simulink model "Trajectory_PID"  (R2024b)
settings: Solver=VariableStepAuto  StartTime=0.0  StopTime=10.0  RelTol=1e-3
libraries: slpidlib x4
settings Model: Creator=GH-X-ST  LastModifiedBy=GH-X-ST

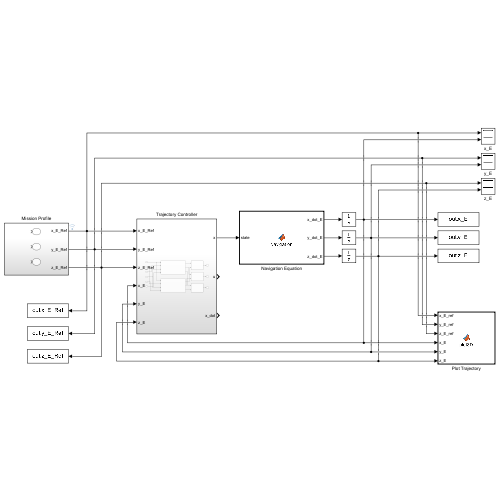
[thumbnail: Simulink's stored preview of the top-level diagram]
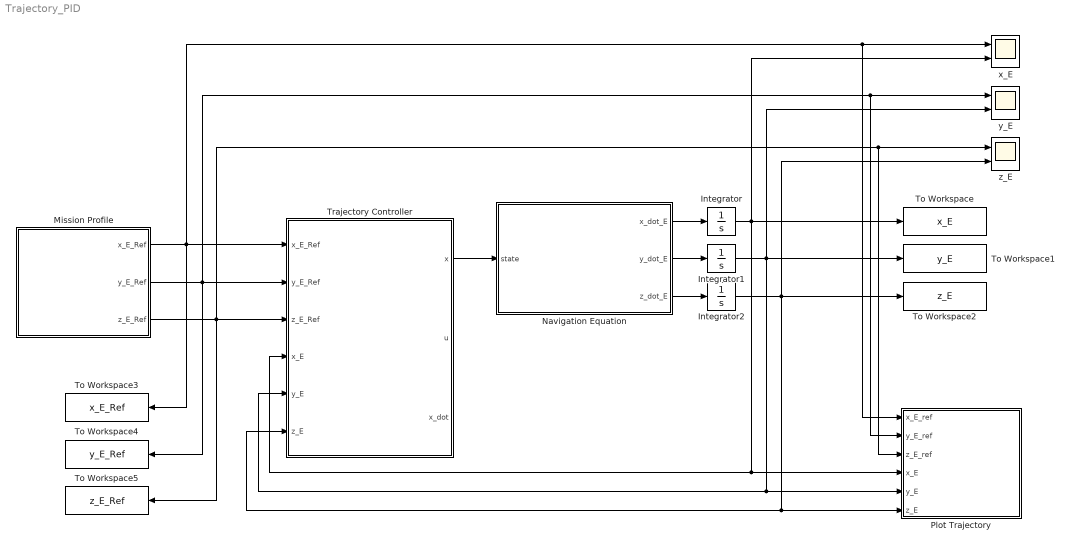
== system Trajectory_PID ==
  Integrator : Integrator
  Integrator1 : Integrator
  Integrator2 : Integrator
  Mission Profile : Subsystem
  Navigation Equation : MATLAB Function  TreatAsAtomicUnit=on
  Plot Trajectory : MATLAB Function  TreatAsAtomicUnit=on
  To Workspace : ToWorkspace  VariableName=x_E  SaveFormat=Timeseries  SampleTime=-1
  To Workspace1 : ToWorkspace  VariableName=y_E  SaveFormat=Timeseries  SampleTime=-1
  To Workspace2 : ToWorkspace  VariableName=z_E  SaveFormat=Timeseries  SampleTime=-1
  To Workspace3 : ToWorkspace  VariableName=x_E_Ref  SaveFormat=Timeseries  SampleTime=-1
  To Workspace4 : ToWorkspace  VariableName=y_E_Ref  SaveFormat=Timeseries  SampleTime=-1
  To Workspace5 : ToWorkspace  VariableName=z_E_Ref  SaveFormat=Timeseries  SampleTime=-1
  Trajectory Controller : Subsystem
  x_E : Scope  NumInputPorts=2
  y_E : Scope  NumInputPorts=2
  z_E : Scope  NumInputPorts=2
  wires:
  Navigation Equation/1(x_dot_E) -> Integrator/1
  Integrator/1 -> Trajectory Controller/4(x_E), Plot Trajectory/4(x_E), x_E/2, To Workspace/1
  Navigation Equation/2(y_dot_E) -> Integrator1/1
  Integrator1/1 -> Trajectory Controller/5(y_E), Plot Trajectory/5(y_E), y_E/2, To Workspace1/1
  Navigation Equation/3(z_dot_E) -> Integrator2/1
  Integrator2/1 -> Trajectory Controller/6(z_E), Plot Trajectory/6(z_E), z_E/2, To Workspace2/1
  Mission Profile/1(x_E_Ref) -> To Workspace3/1, Plot Trajectory/1(x_E_ref), x_E/1, Trajectory Controller/1(x_E_Ref)
  Trajectory Controller/1(x) -> Navigation Equation/1(state)
  Mission Profile/2(y_E_Ref) -> Plot Trajectory/2(y_E_ref), y_E/1, Trajectory Controller/2(y_E_Ref), To Workspace4/1
  Mission Profile/3(z_E_Ref) -> To Workspace5/1, Plot Trajectory/3(z_E_ref), z_E/1, Trajectory Controller/3(z_E_Ref)

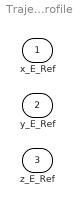
== system Trajectory_PID/Mission Profile ==
  x_E_Ref : Outport
  y_E_Ref : Outport  Port=2
  z_E_Ref : Outport  Port=3

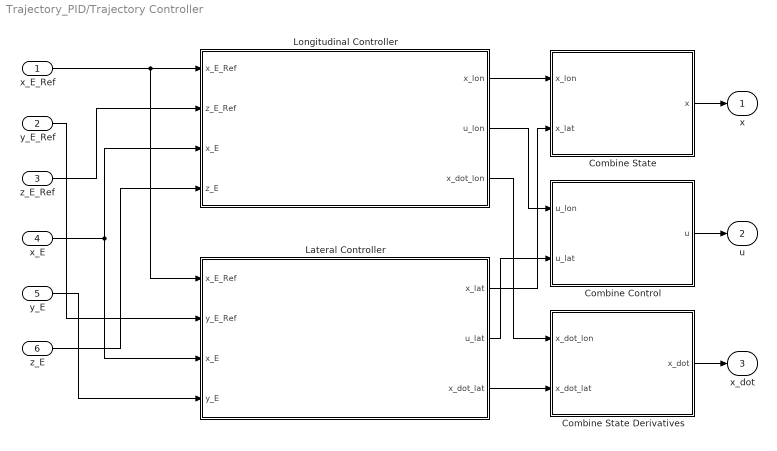
== system Trajectory_PID/Trajectory Controller ==
  x_E_Ref : Inport
  y_E_Ref : Inport  Port=2
  z_E_Ref : Inport  Port=3
  x_E : Inport  Port=4
  y_E : Inport  Port=5
  z_E : Inport  Port=6
  Combine Control : MATLAB Function  TreatAsAtomicUnit=on
  Combine State : MATLAB Function  TreatAsAtomicUnit=on
  Combine State Derivatives : MATLAB Function  TreatAsAtomicUnit=on
  Lateral Controller : Subsystem
  Longitudinal Controller : Subsystem
  x : Outport
  u : Outport  Port=2
  x_dot : Outport  Port=3
  wires:
  Combine State/1(x) -> x/1
  Combine Control/1(u) -> u/1
  Longitudinal Controller/2(u_lon) -> Combine Control/1(u_lon)
  Longitudinal Controller/1(x_lon) -> Combine State/1(x_lon)
  Lateral Controller/1(x_lat) -> Combine State/2(x_lat)
  Lateral Controller/2(u_lat) -> Combine Control/2(u_lat)
  Combine State Derivatives/1(x_dot) -> x_dot/1
  Lateral Controller/3(x_dot_lat) -> Combine State Derivatives/2(x_dot_lat)
  Longitudinal Controller/3(x_dot_lon) -> Combine State Derivatives/1(x_dot_lon)
  x_E_Ref/1 -> Lateral Controller/1(x_E_Ref), Longitudinal Controller/1(x_E_Ref)
  z_E_Ref/1 -> Longitudinal Controller/2(z_E_Ref)
  x_E/1 -> Lateral Controller/3(x_E), Longitudinal Controller/3(x_E)
  z_E/1 -> Longitudinal Controller/4(z_E)
  y_E_Ref/1 -> Lateral Controller/2(y_E_Ref)
  y_E/1 -> Lateral Controller/4(y_E)

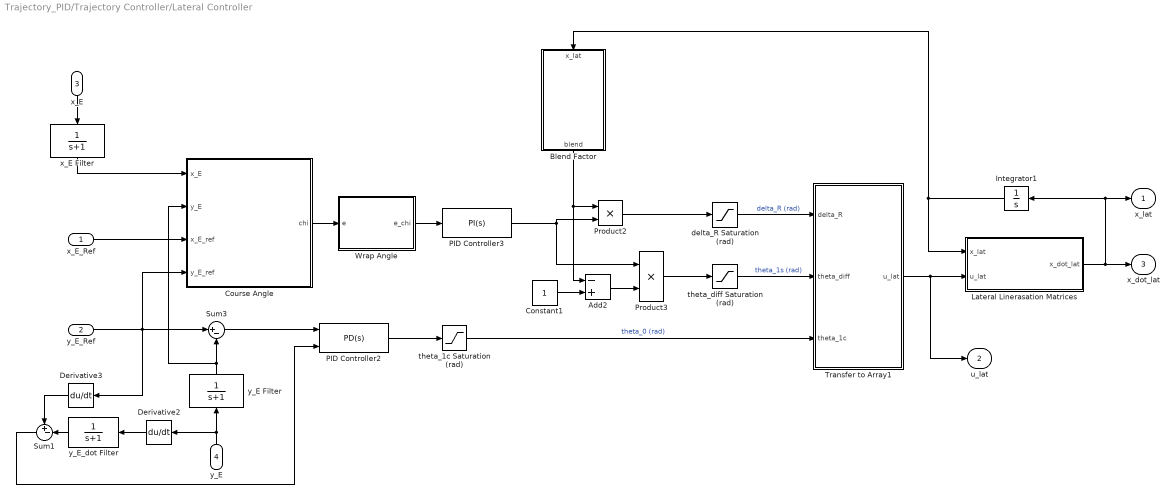
== system Trajectory_PID/Trajectory Controller/Lateral Controller ==
  x_E_Ref : Inport
  y_E_Ref : Inport  Port=2
  x_E : Inport  Port=3
  y_E : Inport  Port=4
  " Course Angle" : MATLAB Function  TreatAsAtomicUnit=on
  Add2 : Sum  Inputs=-+
  Blend Factor : MATLAB Function  TreatAsAtomicUnit=on
  Constant1 : Constant
  Derivative2 : Derivative  CoefficientInTFapproximation=0.05
  Derivative3 : Derivative  CoefficientInTFapproximation=0.05
  Integrator1 : Integrator
  Lateral Linerasation Matrices : MATLAB Function  TreatAsAtomicUnit=on
  PID Controller2 : slpidlib/PID Controller  Controller=PD  Form=Parallel  TimeDomain=Continuous-time  UseExternalTs=off  SampleTime=-1  IntegratorMethod=Forward Euler  FilterMethod=Forward Euler  ControllerParametersSource=internal  P=0.01  I=0.005  UseKiTs=off  D=0.005  UseExternalDerivativeSource=on  N=100  UseFilter=on  TunerSelectOption=Transfer Function Based (PID Tuner App)  InitialConditionSource=internal  InitialConditionForIntegrator=0  InitialConditionForFilter=0  DifferentiatorICPrevScaledInput=0  ExternalReset=none  TrackingMode=off  Kt=1  LimitOutput=on  SatLimitsSource=internal  UpperSaturationLimit=1  LowerSaturationLimit=-1  LinearizeAsGain=on  AntiWindupMode=none  Kb=1  LimitIntegrator=off  UpperIntegratorSaturationLimit=inf  LowerIntegratorSaturationLimit=-inf  POutMin=[]  POutMax=[]  IOutMin=[]  IOutMax=[]  DOutMin=[]  DOutMax=[]  NOutMin=[]  NOutMax=[]  SumOutMin=[]  SumOutMax=[]  SaturationOutMin=[]  SaturationOutMax=[]  PParamMin=[]  PParamMax=[]  IParamMin=[]  IParamMax=[]  DParamMin=[]  DParamMax=[]  NParamMin=[]  NParamMax=[]  KbParamMin=[]  KbParamMax=[]  KtParamMin=[]  KtParamMax=[]  KbOutMin=[]  KbOutMax=[]  KtOutMin=[]  KtOutMax=[]  IntegratorOutMin=[]  IntegratorOutMax=[]  FilterOutMin=[]  FilterOutMax=[]  SumI1OutMin=[]  SumI1OutMax=[]  SumI2OutMin=[]  SumI2OutMax=[]  SumI3OutMin=[]  SumI3OutMax=[]  SumI4OutMin=[]  SumI4OutMax=[]  SumDOutMin=[]  SumDOutMax=[]  DifferentiatorOutMin=[]  DifferentiatorOutMax=[]  FilterDiffOutCoefMin=[]  FilterDiffOutCoefMax=[]  ReciprocalOutMin=[]  ReciprocalOutMax=[]  SumDenOutMin=[]  SumDenOutMax=[]  SumNumOutMin=[]  SumNumOutMax=[]  DivideOutMin=[]  DivideOutMax=[]  UdiffTsProdOutMin=[]  UdiffTsProdOutMax=[]  NTsProdOutMin=[]  NTsProdOutMax=[]  UintegralTsProdOutMin=[]  UintegralTsProdOutMax=[]  UngainTsProdOutMin=[]  UngainTsProdOutMax=[]  ClampingZeroOutDataTypeStr=Inherit: Inherit via back propagation  ClampingZeroOutMin=[]  ClampingZeroOutMax=[]  FilterDenConstantOutDataTypeStr=Inherit: Inherit via back propagation  FilterDenConstantOutMin=[]  FilterDenConstantOutMax=[]  PCopyOutDataTypeStr=Inherit: Inherit via back propagation  PCopyOutMin=[]  PCopyOutMax=[]  NCopyOutDataTypeStr=Inherit: Inherit via back propagation  NCopyOutMin=[]  NCopyOutMax=[]  IntegratorContinuousStateAttributes=''  IntegratorStateMustResolveToSignalObject=off  IntegratorRTWStateStorageClass=Auto  FilterContinuousStateAttributes=''  FilterStateMustResolveToSignalObject=off  FilterRTWStateStorageClass=Auto  ParallelPVariant=InternalParameters  IdealPVariant=Disabled  IVariant=Disabled  DVariant=InternalParameters  IntegratorVariant=Disabled  SatVariant=Enabled  AWVariant=Disabled  PCopyVariant=Disabled  TRVariant=Disabled  FdbkBlocksVariant=Forward  IdealPFdbkVariant=Disabled  SatFdbkVariant=Disabled  DerivativeFilterVariant=ContFilterOnly  NVariant=InternalParameters  NCopyVariant=Disabled  FilterICVariant=InternalICsFilter  IntegratorICVariant=Disabled  ExternalResetVariant=Disabled  TRSumVariant=Passthrough  SumFdbkVariant=Disabled  SumVariant=Sum_PD  TsampFilterVariant=InternalTs  TsampNgainVariant=Passthrough  TsampIntegralVariant=Disabled_SignalSpec  ExternalSaturationOutDataTypeStr=Inherit: Same as second input  DerivativeSourceVariant=ExternalYdot  PreIntVariant=InternalPreInt
  PID Controller3 : slpidlib/PID Controller  Controller=PI  Form=Parallel  TimeDomain=Continuous-time  UseExternalTs=off  SampleTime=-1  IntegratorMethod=Forward Euler  FilterMethod=Forward Euler  ControllerParametersSource=internal  P=0.01  I=0.005  UseKiTs=off  D=0.005  UseExternalDerivativeSource=off  N=100  UseFilter=on  TunerSelectOption=Transfer Function Based (PID Tuner App)  InitialConditionSource=internal  InitialConditionForIntegrator=0  InitialConditionForFilter=0  DifferentiatorICPrevScaledInput=0  ExternalReset=none  TrackingMode=off  Kt=1  LimitOutput=on  SatLimitsSource=internal  UpperSaturationLimit=1  LowerSaturationLimit=-1  LinearizeAsGain=on  AntiWindupMode=none  Kb=1  LimitIntegrator=off  UpperIntegratorSaturationLimit=inf  LowerIntegratorSaturationLimit=-inf  POutMin=[]  POutMax=[]  IOutMin=[]  IOutMax=[]  DOutMin=[]  DOutMax=[]  NOutMin=[]  NOutMax=[]  SumOutMin=[]  SumOutMax=[]  SaturationOutMin=[]  SaturationOutMax=[]  PParamMin=[]  PParamMax=[]  IParamMin=[]  IParamMax=[]  DParamMin=[]  DParamMax=[]  NParamMin=[]  NParamMax=[]  KbParamMin=[]  KbParamMax=[]  KtParamMin=[]  KtParamMax=[]  KbOutMin=[]  KbOutMax=[]  KtOutMin=[]  KtOutMax=[]  IntegratorOutMin=[]  IntegratorOutMax=[]  FilterOutMin=[]  FilterOutMax=[]  SumI1OutMin=[]  SumI1OutMax=[]  SumI2OutMin=[]  SumI2OutMax=[]  SumI3OutMin=[]  SumI3OutMax=[]  SumI4OutMin=[]  SumI4OutMax=[]  SumDOutMin=[]  SumDOutMax=[]  DifferentiatorOutMin=[]  DifferentiatorOutMax=[]  FilterDiffOutCoefMin=[]  FilterDiffOutCoefMax=[]  ReciprocalOutMin=[]  ReciprocalOutMax=[]  SumDenOutMin=[]  SumDenOutMax=[]  SumNumOutMin=[]  SumNumOutMax=[]  DivideOutMin=[]  DivideOutMax=[]  UdiffTsProdOutMin=[]  UdiffTsProdOutMax=[]  NTsProdOutMin=[]  NTsProdOutMax=[]  UintegralTsProdOutMin=[]  UintegralTsProdOutMax=[]  UngainTsProdOutMin=[]  UngainTsProdOutMax=[]  ClampingZeroOutDataTypeStr=Inherit: Inherit via back propagation  ClampingZeroOutMin=[]  ClampingZeroOutMax=[]  FilterDenConstantOutDataTypeStr=Inherit: Inherit via back propagation  FilterDenConstantOutMin=[]  FilterDenConstantOutMax=[]  PCopyOutDataTypeStr=Inherit: Inherit via back propagation  PCopyOutMin=[]  PCopyOutMax=[]  NCopyOutDataTypeStr=Inherit: Inherit via back propagation  NCopyOutMin=[]  NCopyOutMax=[]  IntegratorContinuousStateAttributes=''  IntegratorStateMustResolveToSignalObject=off  IntegratorRTWStateStorageClass=Auto  FilterContinuousStateAttributes=''  FilterStateMustResolveToSignalObject=off  FilterRTWStateStorageClass=Auto  ParallelPVariant=InternalParameters  IdealPVariant=Disabled  IVariant=InternalParameters  DVariant=Disabled  IntegratorVariant=Continuous  SatVariant=Enabled  AWVariant=Passthrough  PCopyVariant=Disabled  TRVariant=Disabled  FdbkBlocksVariant=Forward  IdealPFdbkVariant=Disabled  SatFdbkVariant=Disabled  DerivativeFilterVariant=Disabled  NVariant=Disabled  NCopyVariant=Disabled_SignalSpec  FilterICVariant=Disabled  IntegratorICVariant=InternalICs  ExternalResetVariant=Disabled  TRSumVariant=Passthrough  SumFdbkVariant=Disabled  SumVariant=Sum_PI  TsampFilterVariant=InternalTs  TsampNgainVariant=Passthrough  TsampIntegralVariant=Disabled_SignalSpec  ExternalSaturationOutDataTypeStr=Inherit: Same as second input  DerivativeSourceVariant=Disabled  PreIntVariant=InternalPreInt
  Product2 : Product
  Product3 : Product
  Sum1 : Sum  Inputs=+-|
  Sum3 : Sum  Inputs=|+-
  Transfer to Array1 : MATLAB Function  TreatAsAtomicUnit=on
  Wrap Angle : MATLAB Function  TreatAsAtomicUnit=on
  delta_R Saturation (rad) : Saturate
  theta_1c Saturation (rad) : Saturate
  theta_diff Saturation (rad) : Saturate
  x_E Filter : TransferFcn  Denominator=[1 1]
  y_E Filter : TransferFcn  Denominator=[1 1]
  y_E_dot Filter : TransferFcn  Denominator=[1 1]
  x_lat : Outport
  u_lat : Outport  Port=2
  x_dot_lat : Outport  Port=3
  wires:
  y_E/1 -> y_E Filter/1, Derivative2/1
  y_E Filter/1 -> Sum3/2, " Course Angle"/2(y_E)
  y_E_Ref/1 -> Derivative3/1, " Course Angle"/4(y_E_ref), Sum3/1
  Sum3/1 -> PID Controller2/1
  PID Controller2/1 -> theta_1c Saturation (rad)/1
  theta_1c Saturation (rad)/1 -> Transfer to Array1/3(theta_1c)  "theta_0 (rad)"
  Transfer to Array1/1(u_lat) -> u_lat/1, Lateral Linerasation Matrices/2(u_lat)
  Lateral Linerasation Matrices/1(x_dot_lat) -> Integrator1/1, x_lat/1, x_dot_lat/1
  Integrator1/1 -> Lateral Linerasation Matrices/1(x_lat), Blend Factor/1(x_lat)
  x_E_Ref/1 -> " Course Angle"/3(x_E_ref)
  " Course Angle"/1(chi) -> Wrap Angle/1(e)
  Wrap Angle/1(e_chi) -> PID Controller3/1
  PID Controller3/1 -> Product2/2, Product3/1
  Blend Factor/1(blend) -> Add2/1, Product2/1
  Constant1/1 -> Add2/2
  Add2/1 -> Product3/2
  Product3/1 -> theta_diff Saturation (rad)/1
  theta_diff Saturation (rad)/1 -> Transfer to Array1/2(theta_diff)  "theta_1s (rad)"
  Product2/1 -> delta_R Saturation (rad)/1
  delta_R Saturation (rad)/1 -> Transfer to Array1/1(delta_R)  "delta_R (rad)"
  x_E/1 -> x_E Filter/1
  x_E Filter/1 -> " Course Angle"/1(x_E)
  Derivative2/1 -> y_E_dot Filter/1
  Derivative3/1 -> Sum1/1
  y_E_dot Filter/1 -> Sum1/2
  Sum1/1 -> PID Controller2/2

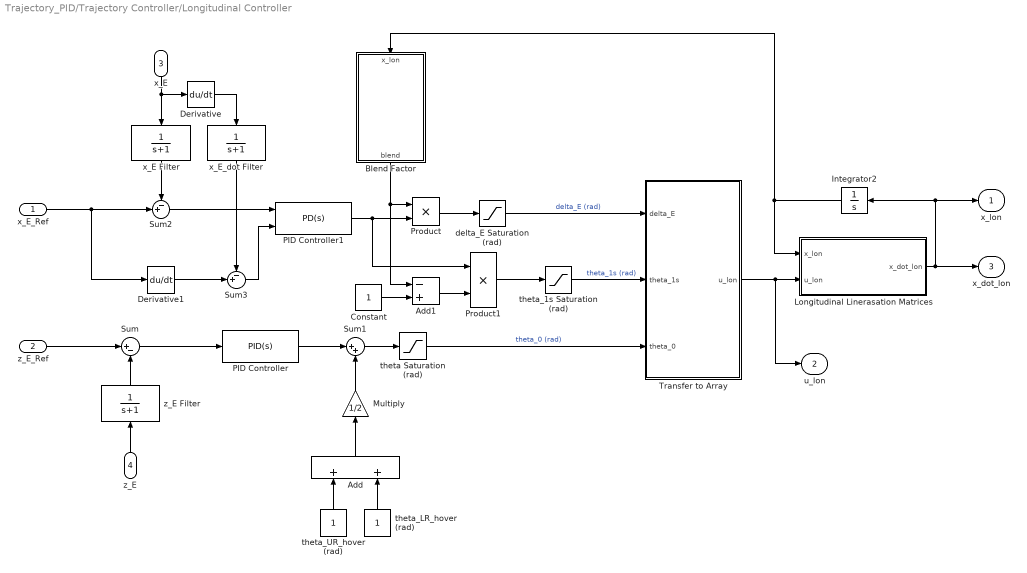
== system Trajectory_PID/Trajectory Controller/Longitudinal Controller ==
  x_E_Ref : Inport
  z_E_Ref : Inport  Port=2
  x_E : Inport  Port=3
  z_E : Inport  Port=4
  Add : Sum
  Add1 : Sum  Inputs=-+
  Blend Factor : MATLAB Function  TreatAsAtomicUnit=on
  Constant : Constant
  Derivative : Derivative  CoefficientInTFapproximation=0.05
  Derivative1 : Derivative  CoefficientInTFapproximation=0.05
  Integrator2 : Integrator
  Longitudinal Linerasation Matrices : MATLAB Function  TreatAsAtomicUnit=on
  Multiply : Gain  Gain=1/2
  PID Controller : slpidlib/PID Controller  Controller=PID  Form=Parallel  TimeDomain=Continuous-time  UseExternalTs=off  SampleTime=-1  IntegratorMethod=Forward Euler  FilterMethod=Forward Euler  ControllerParametersSource=internal  P=0.01  I=0.005  UseKiTs=off  D=0.005  UseExternalDerivativeSource=off  N=100  UseFilter=on  TunerSelectOption=Transfer Function Based (PID Tuner App)  InitialConditionSource=internal  InitialConditionForIntegrator=0  InitialConditionForFilter=0  DifferentiatorICPrevScaledInput=0  ExternalReset=none  TrackingMode=off  Kt=1  LimitOutput=on  SatLimitsSource=internal  UpperSaturationLimit=1  LowerSaturationLimit=-1  LinearizeAsGain=on  AntiWindupMode=none  Kb=1  LimitIntegrator=off  UpperIntegratorSaturationLimit=inf  LowerIntegratorSaturationLimit=-inf  POutMin=[]  POutMax=[]  IOutMin=[]  IOutMax=[]  DOutMin=[]  DOutMax=[]  NOutMin=[]  NOutMax=[]  SumOutMin=[]  SumOutMax=[]  SaturationOutMin=[]  SaturationOutMax=[]  PParamMin=[]  PParamMax=[]  IParamMin=[]  IParamMax=[]  DParamMin=[]  DParamMax=[]  NParamMin=[]  NParamMax=[]  KbParamMin=[]  KbParamMax=[]  KtParamMin=[]  KtParamMax=[]  KbOutMin=[]  KbOutMax=[]  KtOutMin=[]  KtOutMax=[]  IntegratorOutMin=[]  IntegratorOutMax=[]  FilterOutMin=[]  FilterOutMax=[]  SumI1OutMin=[]  SumI1OutMax=[]  SumI2OutMin=[]  SumI2OutMax=[]  SumI3OutMin=[]  SumI3OutMax=[]  SumI4OutMin=[]  SumI4OutMax=[]  SumDOutMin=[]  SumDOutMax=[]  DifferentiatorOutMin=[]  DifferentiatorOutMax=[]  FilterDiffOutCoefMin=[]  FilterDiffOutCoefMax=[]  ReciprocalOutMin=[]  ReciprocalOutMax=[]  SumDenOutMin=[]  SumDenOutMax=[]  SumNumOutMin=[]  SumNumOutMax=[]  DivideOutMin=[]  DivideOutMax=[]  UdiffTsProdOutMin=[]  UdiffTsProdOutMax=[]  NTsProdOutMin=[]  NTsProdOutMax=[]  UintegralTsProdOutMin=[]  UintegralTsProdOutMax=[]  UngainTsProdOutMin=[]  UngainTsProdOutMax=[]  ClampingZeroOutDataTypeStr=Inherit: Inherit via back propagation  ClampingZeroOutMin=[]  ClampingZeroOutMax=[]  FilterDenConstantOutDataTypeStr=Inherit: Inherit via back propagation  FilterDenConstantOutMin=[]  FilterDenConstantOutMax=[]  PCopyOutDataTypeStr=Inherit: Inherit via back propagation  PCopyOutMin=[]  PCopyOutMax=[]  NCopyOutDataTypeStr=Inherit: Inherit via back propagation  NCopyOutMin=[]  NCopyOutMax=[]  IntegratorContinuousStateAttributes=''  IntegratorStateMustResolveToSignalObject=off  IntegratorRTWStateStorageClass=Auto  FilterContinuousStateAttributes=''  FilterStateMustResolveToSignalObject=off  FilterRTWStateStorageClass=Auto  ParallelPVariant=InternalParameters  IdealPVariant=Disabled  IVariant=InternalParameters  DVariant=InternalParameters  IntegratorVariant=Continuous  SatVariant=Enabled  AWVariant=Passthrough  PCopyVariant=Disabled  TRVariant=Disabled  FdbkBlocksVariant=Forward  IdealPFdbkVariant=Disabled  SatFdbkVariant=Disabled  DerivativeFilterVariant=ContFilter  NVariant=InternalParameters  NCopyVariant=Disabled  FilterICVariant=InternalICsFilter  IntegratorICVariant=InternalICs  ExternalResetVariant=Disabled  TRSumVariant=Passthrough  SumFdbkVariant=Disabled  SumVariant=Sum_PID  TsampFilterVariant=InternalTs  TsampNgainVariant=Passthrough  TsampIntegralVariant=Disabled_SignalSpec  ExternalSaturationOutDataTypeStr=Inherit: Same as second input  DerivativeSourceVariant=ErrorSignal  PreIntVariant=InternalPreInt
  PID Controller1 : slpidlib/PID Controller  Controller=PD  Form=Parallel  TimeDomain=Continuous-time  UseExternalTs=off  SampleTime=-1  IntegratorMethod=Forward Euler  FilterMethod=Forward Euler  ControllerParametersSource=internal  P=0.01  I=0.005  UseKiTs=off  D=0.005  UseExternalDerivativeSource=on  N=100  UseFilter=on  TunerSelectOption=Transfer Function Based (PID Tuner App)  InitialConditionSource=internal  InitialConditionForIntegrator=0  InitialConditionForFilter=0  DifferentiatorICPrevScaledInput=0  ExternalReset=none  TrackingMode=off  Kt=1  LimitOutput=on  SatLimitsSource=internal  UpperSaturationLimit=1  LowerSaturationLimit=-1  LinearizeAsGain=on  AntiWindupMode=none  Kb=1  LimitIntegrator=off  UpperIntegratorSaturationLimit=inf  LowerIntegratorSaturationLimit=-inf  POutMin=[]  POutMax=[]  IOutMin=[]  IOutMax=[]  DOutMin=[]  DOutMax=[]  NOutMin=[]  NOutMax=[]  SumOutMin=[]  SumOutMax=[]  SaturationOutMin=[]  SaturationOutMax=[]  PParamMin=[]  PParamMax=[]  IParamMin=[]  IParamMax=[]  DParamMin=[]  DParamMax=[]  NParamMin=[]  NParamMax=[]  KbParamMin=[]  KbParamMax=[]  KtParamMin=[]  KtParamMax=[]  KbOutMin=[]  KbOutMax=[]  KtOutMin=[]  KtOutMax=[]  IntegratorOutMin=[]  IntegratorOutMax=[]  FilterOutMin=[]  FilterOutMax=[]  SumI1OutMin=[]  SumI1OutMax=[]  SumI2OutMin=[]  SumI2OutMax=[]  SumI3OutMin=[]  SumI3OutMax=[]  SumI4OutMin=[]  SumI4OutMax=[]  SumDOutMin=[]  SumDOutMax=[]  DifferentiatorOutMin=[]  DifferentiatorOutMax=[]  FilterDiffOutCoefMin=[]  FilterDiffOutCoefMax=[]  ReciprocalOutMin=[]  ReciprocalOutMax=[]  SumDenOutMin=[]  SumDenOutMax=[]  SumNumOutMin=[]  SumNumOutMax=[]  DivideOutMin=[]  DivideOutMax=[]  UdiffTsProdOutMin=[]  UdiffTsProdOutMax=[]  NTsProdOutMin=[]  NTsProdOutMax=[]  UintegralTsProdOutMin=[]  UintegralTsProdOutMax=[]  UngainTsProdOutMin=[]  UngainTsProdOutMax=[]  ClampingZeroOutDataTypeStr=Inherit: Inherit via back propagation  ClampingZeroOutMin=[]  ClampingZeroOutMax=[]  FilterDenConstantOutDataTypeStr=Inherit: Inherit via back propagation  FilterDenConstantOutMin=[]  FilterDenConstantOutMax=[]  PCopyOutDataTypeStr=Inherit: Inherit via back propagation  PCopyOutMin=[]  PCopyOutMax=[]  NCopyOutDataTypeStr=Inherit: Inherit via back propagation  NCopyOutMin=[]  NCopyOutMax=[]  IntegratorContinuousStateAttributes=''  IntegratorStateMustResolveToSignalObject=off  IntegratorRTWStateStorageClass=Auto  FilterContinuousStateAttributes=''  FilterStateMustResolveToSignalObject=off  FilterRTWStateStorageClass=Auto  ParallelPVariant=InternalParameters  IdealPVariant=Disabled  IVariant=Disabled  DVariant=InternalParameters  IntegratorVariant=Disabled  SatVariant=Enabled  AWVariant=Disabled  PCopyVariant=Disabled  TRVariant=Disabled  FdbkBlocksVariant=Forward  IdealPFdbkVariant=Disabled  SatFdbkVariant=Disabled  DerivativeFilterVariant=ContFilterOnly  NVariant=InternalParameters  NCopyVariant=Disabled  FilterICVariant=InternalICsFilter  IntegratorICVariant=Disabled  ExternalResetVariant=Disabled  TRSumVariant=Passthrough  SumFdbkVariant=Disabled  SumVariant=Sum_PD  TsampFilterVariant=InternalTs  TsampNgainVariant=Passthrough  TsampIntegralVariant=Disabled_SignalSpec  ExternalSaturationOutDataTypeStr=Inherit: Same as second input  DerivativeSourceVariant=ExternalYdot  PreIntVariant=InternalPreInt
  Product : Product
  Product1 : Product
  Sum : Sum  Inputs=|+-
  Sum1 : Sum  Inputs=|++
  Sum2 : Sum  Inputs=-+|
  Sum3 : Sum  Inputs=-+|
  Transfer to Array : MATLAB Function  TreatAsAtomicUnit=on
  delta_E Saturation (rad) : Saturate
  theta Saturation (rad) : Saturate
  theta_1s Saturation (rad) : Saturate
  theta_LR_hover (rad) : Constant
  theta_UR_hover (rad) : Constant
  x_E Filter : TransferFcn  Denominator=[1 1]
  x_E_dot Filter : TransferFcn  Denominator=[1 1]
  z_E Filter : TransferFcn  Denominator=[1 1]
  x_lon : Outport
  u_lon : Outport  Port=2
  x_dot_lon : Outport  Port=3
  wires:
  z_E_Ref/1 -> Sum/1
  Sum/1 -> PID Controller/1
  PID Controller/1 -> Sum1/1
  Sum1/1 -> theta Saturation (rad)/1
  theta_UR_hover (rad)/1 -> Add/1
  theta_LR_hover (rad)/1 -> Add/2
  Multiply/1 -> Sum1/2
  Add/1 -> Multiply/1
  theta Saturation (rad)/1 -> Transfer to Array/3(theta_0)  "theta_0 (rad)"
  z_E Filter/1 -> Sum/2
  z_E/1 -> z_E Filter/1
  x_E/1 -> Derivative/1, x_E Filter/1
  x_E_Ref/1 -> Derivative1/1, Sum2/2
  Sum2/1 -> PID Controller1/1
  Integrator2/1 -> Longitudinal Linerasation Matrices/1(x_lon), Blend Factor/1(x_lon)
  Longitudinal Linerasation Matrices/1(x_dot_lon) -> Integrator2/1, x_lon/1, x_dot_lon/1
  Blend Factor/1(blend) -> Add1/1, Product/1
  PID Controller1/1 -> Product1/1, Product/2
  Product/1 -> delta_E Saturation (rad)/1
  delta_E Saturation (rad)/1 -> Transfer to Array/1(delta_E)  "delta_E (rad)"
  Constant/1 -> Add1/2
  Add1/1 -> Product1/2
  Product1/1 -> theta_1s Saturation (rad)/1
  theta_1s Saturation (rad)/1 -> Transfer to Array/2(theta_1s)  "theta_1s (rad)"
  Transfer to Array/1(u_lon) -> u_lon/1, Longitudinal Linerasation Matrices/2(u_lon)
  Derivative/1 -> x_E_dot Filter/1
  x_E Filter/1 -> Sum2/1
  Derivative1/1 -> Sum3/2
  x_E_dot Filter/1 -> Sum3/1
  Sum3/1 -> PID Controller1/2

== matlab function Trajectory_PID/Trajectory Controller/Lateral Controller/Lateral Linerasation Matrices ==
  data: x_dot_lat output; x_lat input; u_lat input
function x_dot_lat = Lon_linear(x_lat, u_lat)
% Author:
%   Hanchen Li (hl3422@ic.ac.uk)
%
% Inputs:
%   x_lat     - [v, p, r, phi, psi]
%   v         - Lateral velocity (m/s)
%   p         - Roll rate (rad/s)
%   r         - Yaw rate (rad/s)
%   phi       - Euler roll angle (rad)
%   psi       - Euler yaw angle (rad)
%
%   u_lat      - [theta_diff, theta_1c, delta_R]
%   theta_diff - Rotor collective difference (rad)
%   theta_1c   - Lateral cyclic (rad)
%   delta_R    - Rudder deflection (rad)
%
% Outputs:
%   x_dot_lat     - [v_dot, p_dot, r_dot, phi_dot, psi_dot]

%% 0 Extract Parameters
v          = x_lat(1);
p          = x_lat(2);
r          = x_lat(3);
phi        = x_lat(4);
psi        = x_lat(5);

theta_diff = u_lat(1);
theta_1c   = u_lat(2);
delta_R    = u_lat(3);

%% 1 Decide blend factor

if v = 0

    x_dot_lat = ;

else
    
    x_dot_lat = ;

end

end

== matlab function Trajectory_PID/Trajectory Controller/Lateral Controller/Blend Factor ==
  data: blend output; x_lat input
function blend = Blend_yaw(x_lat)
% Author:
%   Hanchen Li (hl3422@ic.ac.uk)
%
% Inputs:
%   x_lat     - [v, p, r, phi, psi]
%   v         - Lateral velocity (m/s)
%   p         - Roll rate (rad/s)
%   r         - Yaw rate (rad/s)
%   phi       - Euler roll angle (rad)
%   psi       - Euler yaw angle (rad)
%
% Outputs:
%   blend     - blend factor

%% 0 Extract Parameters

v   = x_lat(1);
p   = x_lat(2);
r   = x_lat(3);
phi = x_lat(4);
psi = x_lat(5);

%% 1 Decide blend factor

if abs(v) < 1e-4

    blend = 0;

elseif abs(v) < 20

    blend = u / 20;

else

    blend = 1;

end

end

== matlab function Trajectory_PID/Trajectory Controller/Lateral Controller/Wrap Angle ==
  data: e_chi output; e input
function e_chi = Wrap_Pi(e)
% Author:
%   Hanchen Li (hl3422@ic.ac.uk)
%
% Inputs:
%   chi
%
% Outputs:
%   e_chi

e_chi = mod(chi + pi, 2 * pi) - pi;

end

== matlab function Trajectory_PID/Plot Trajectory ==
  data: x_E_ref input; y_E_ref input; z_E_ref input; x_E input; y_E input; z_E input
function plot3D(x_E_ref, y_E_ref, z_E_ref, x_E, y_E, z_E)
% Author:
%   Hanchen Li (hl3422@ic.ac.uk)
%
% Inputs:
%   x_E_ref   - Distance in the Earth x-direction (m/s)
%   x_E_ref   - Distance in the Earth x-direction (m/s)
%   x_E_ref   - Distance in the Earth x-direction (m/s)
%   x_E       - Distance in the Earth x-direction (m/s)
%   x_E       - Distance in the Earth x-direction (m/s)
%   x_E       - Distance in the Earth x-direction (m/s)
%
% Outputs:
%   Real time 3D trajectory plot

% Persistent line objects for plotting
persistent refLine actLine firstRun

% Initialization (on first call)
if isempty(firstRun)
    
    figure(1); clf;
    refLine = animatedline('Color', [0/255 0/255 128/255], 'LineStyle', '--', 'LineWidth', 1.5, 'DisplayName', 'Reference');
    actLine = animatedline('Color', [220/255 20/255 60/255], 'LineStyle', '-',  'LineWidth', 1.5, 'DisplayName', 'Actual');
    xlabel('x_E'); ylabel('y_E'); zlabel('z_E');
    title('HALO 3-D trajectory plot.');
    grid on;
    view(3);
    legend show;
    axis equal;
    hold on;
    firstRun = true;
end

% Add new points
addpoints(refLine, x_ref, y_ref, z_ref);
addpoints(actLine, x, y, z);
    
% Update plot
drawnow limitrate;

end

== matlab function Trajectory_PID/Navigation Equation ==
  data: x_dot_E output; y_dot_E output; z_dot_E output; state input
function [x_dot_E, y_dot_E, z_dot_E] = Navigation(state)
% Author:
%   Hanchen Li (hl3422@ic.ac.uk)
%
% Inputs:
%   state     - [u, v, w, p, q, r, phi, theta, psi]
%   u         - Forward velocity (m/s)
%   v         - Lateral velocity (m/s)
%   w         - Vertical velocity (m/s)
%   p         - Roll rate (rad/s)
%   q         - Pitch rate (rad/s)
%   r         - Yaw rate (rad/s)
%   phi       - Euler roll angle (rad)
%   theta     - Euler pitch angle (rad)
%   psi       - Euler yaw angle (rad)
%
% Outputs:
%   x_dot_E   - Velocity in the Earth x-direction (m/s)
%   y_dot_E   - Velocity in the Earth y-direction (m/s)
%   z_dot_E   - Velocity in the Earth z-direction (m/s)

%% 0 Basic Parameters

% 0.1 Extract parameters
% state - [u, v, w, p, q, r, phi, theta, psi]
u = state(1);
v = state(2);
w = state(3);
p = state(4);
q = state(5);
r = state(6);
phi = state(7);
theta = state(8);
psi = state(9);

% 0.2 Compute trigonometric values
cphi = cos(phi);
sphi = sin(phi);
ctheta = cos(theta);
stheta = sin(theta);
cpsi = cos(psi);
spsi = sin(psi);

% 0.3 Transformation matrix from body to inertial frame
T = [...
     ctheta * cpsi, sphi * stheta * cpsi - cphi * spsi, cphi * stheta * cpsi + sphi * spsi;
     ctheta * spsi, sphi * stheta * spsi + cphi * cpsi, cphi * stheta * spsi - sphi * cpsi;
     -stheta      , sphi * ctheta                     , cphi * ctheta];

%% 1 Calculation
% 1.1 Body velocity vector
V_body = [u; v; w];

% 1.2 Compute inertial velocity
V_inertial = T * V_body;

% 1.3 Output
x_dot_E = V_inertial(1);
y_dot_E = V_inertial(2);
z_dot_E = V_inertial(3);

end

== matlab function Trajectory_PID/Trajectory Controller/Combine State ==
  data: x output; x_lon input; x_lat input
function x = Combine_State(x_lon, x_lat)
% Author:
%   Hanchen Li (hl3422@ic.ac.uk)
%
% Inputs:
%   x_lon     - [u, w, q, theta]
%   u         - Forward velocity (m/s)
%   w         - Vertical velocity (m/s)
%   q         - Pitch rate (rad/s)
%   theta     - Euler pitch angle (rad)
%
%   x_lat     - [v, p, r, phi, psi]
%   v         - Lateral velocity (m/s)
%   p         - Roll rate (rad/s)
%   r         - Yaw rate (rad/s)
%   phi       - Euler roll angle (rad)
%   psi       - Euler yaw angle (rad)
%
% Outputs:
%   x         - [u, v, w, p, q, r, phi, theta, psi]
%   u         - Forward velocity (m/s)
%   v         - Lateral velocity (m/s)
%   w         - Vertical velocity (m/s)
%   p         - Roll rate (rad/s)
%   q         - Pitch rate (rad/s)
%   r         - Yaw rate (rad/s)
%   phi       - Euler roll angle (rad)
%   theta     - Euler pitch angle (rad)
%   psi       - Euler yaw angle (rad)

%% 0 Extract Parameters

% x_lon - [u, w, q, theta]
u     = x_lon(1);
w     = x_lon(2);
q     = x_lon(3);
theta = x_lon(4);

% x_lat - [v, p, r, phi, psi]
v     = x_lat(1);
p     = x_lat(2);
r     = x_lat(3);
phi   = x_lat(4);
psi   = x_lat(5);

%% 1 Combination

x = [u, v, w, p, q, r, phi, theta, psi];

end

== matlab function Trajectory_PID/Trajectory Controller/Combine Control ==
  data: u output; u_lon input; u_lat input
function u = Combine_Control(u_lon, u_lat)
% Author:
%   Hanchen Li (hl3422@ic.ac.uk)
%
% Inputs:
%   u_lon      - [theta_0, theta_1s, delta_E]
%   theta_0    - Average rotor collective (rad)
%   theta_1s   - Longitudinal cyclic (rad)
%   delta_E    - Elevator deflection (rad)
%
%   u_lat      - [theta_diff, theta_1c, delta_R]
%   theta_diff - Rotor collective difference (rad)
%   theta_1c   - Lateral cyclic (rad)
%   delta_R    - Rudder deflection (rad)
%
% Outputs:
%   u          - [theta_LR, theta_UR, theta_1s, theta_1c, delta_E, delta_R]
%   theta_LR   - Lower rotor collective (rad)
%   theta_UR   - Upper rotor collective (rad)
%   theta_1s   - Longitudinal cyclic (rad)
%   theta_1c   - Lateral cyclic (rad)
%   delta_E    - Elevator deflection (rad)
%   delta_R    - Rudder deflection (rad)

%% 0 Extract Parameters

% u_lon - [theta_0, theta_1s, delta_E]
theta_0    = u_lon(1);
theta_1s   = u_lon(2);
delta_E    = u_lon(3);

% u_lat - [theta_diff, theta_1c, delta_R]
theta_diff = u_lat(1);
theta_1c   = u_lat(2);
delta_R    = u_lat(3);

%% 1 Combination

theta_LR = theta_0 - theta_diff / 2;

theta_UR = theta_0 + theta_diff / 2;

u = [theta_LR, theta_UR, theta_1s, theta_1c, delta_E, delta_R];

end

== matlab function Trajectory_PID/Trajectory Controller/Combine State Derivatives ==
  data: x_dot output; x_dot_lon input; x_dot_lat input
function x_dot = Combine_State(x_dot_lon, x_dot_lat)
% Author:
%   Hanchen Li (hl3422@ic.ac.uk)
%
% Inputs:
%   x_lon     - [u, w, q, theta]
%   u         - Forward velocity (m/s)
%   w         - Vertical velocity (m/s)
%   q         - Pitch rate (rad/s)
%   theta     - Euler pitch angle (rad)
%
%   x_lat     - [v, p, r, phi, psi]
%   v         - Lateral velocity (m/s)
%   p         - Roll rate (rad/s)
%   r         - Yaw rate (rad/s)
%   phi       - Euler roll angle (rad)
%   psi       - Euler yaw angle (rad)
%
% Outputs:
%   x         - [u, v, w, p, q, r, phi, theta, psi]
%   u         - Forward velocity (m/s)
%   v         - Lateral velocity (m/s)
%   w         - Vertical velocity (m/s)
%   p         - Roll rate (rad/s)
%   q         - Pitch rate (rad/s)
%   r         - Yaw rate (rad/s)
%   phi       - Euler roll angle (rad)
%   theta     - Euler pitch angle (rad)
%   psi       - Euler yaw angle (rad)

%% 0 Extract Parameters

% x_lon - [u, w, q, theta]
u_dot     = x_dot_lon(1);
w_dot     = x_dot_lon(2);
q_dot     = x_dot_lon(3);
theta_dot = x_dot_lon(4);

% x_lat - [v, p, r, phi, psi]
v_dot     = x_dot_lat(1);
p_dot     = x_dot_lat(2);
r_dot     = x_dot_lat(3);
phi_dot   = x_dot_lat(4);
psi_dot   = x_dot_lat(5);

%% 1 Combination

x_dot = [u_dot, v_dot, w_dot, p_dot, q_dot, r_dot, phi_dot, theta_dot, psi_dot];

end

== matlab function Trajectory_PID/Trajectory Controller/Longitudinal Controller/Blend Factor ==
  data: blend output; x_lon input
function blend = Blend_pitch(x_lon)
% Author:
%   Hanchen Li (hl3422@ic.ac.uk)
%
% Inputs:
%   x_lon     - [u, w, q, theta]
%   u         - Forward velocity (m/s)
%   w         - Vertical velocity (m/s)
%   q         - Pitch rate (rad/s)
%   theta     - Euler pitch angle (rad)
%
% Outputs:
%   blend     - blend factor

%% 0 Extract Parameters

u     = x_lon(1);
w     = x_lon(2);
q     = x_lon(3);
theta = x_lon(4);

%% 1 Decide blend factor

if abs(u) < 1e-4

    blend = 0;

elseif abs(u) < 110

    blend = u / 110;

else

    blend = 1;

end

end

== matlab function Trajectory_PID/Trajectory Controller/Longitudinal Controller/Longitudinal Linerasation Matrices ==
  data: x_dot_lon output; x_lon input; u_lon input
function x_dot_lon = Lon_linear(x_lon, u_lon)
% Author:
%   Hanchen Li (hl3422@ic.ac.uk)
%
% Inputs:
%   x_lon     - [u, w, q, theta]
%   u         - Forward velocity (m/s)
%   w         - Vertical velocity (m/s)
%   q         - Pitch rate (rad/s)
%   theta     - Euler pitch angle (rad)
%
%   u_lon     - [theta_0, theta_1s, delta_E]
%   theta_0   - Average rotor collective (rad)
%   theta_1s  - Longitudinal cyclic (rad)
%   delta_E   - Elevator deflection (rad)
%
% Outputs:
%   x_dot_lon - [u_dot, w_dot, q_dot, theta_dot]

%% 0 Extract Parameters
u     = x_lon(1);
w     = x_lon(2);
q     = x_lon(3);
theta = x_lon(4);

theta_0 = u_lon(1);
theta_1s = u_lon(2);
delta_E = u_lon(3);

%% 1 Decide blend factor

if u = 0

    x_dot_lon = ;

else
    
    x_dot_lon = ;

end

end

== matlab function Trajectory_PID/Trajectory Controller/Longitudinal Controller/Transfer to Array ==
  data: delta_E input; u_lon output; theta_1s input; theta_0 input
function u_lon = u_lon_form(delta_E, theta_1s, theta_0)
% Author:
%   Hanchen Li (hl3422@ic.ac.uk)
%
% Inputs:
%   theta_0   - Average rotor collective (rad)
%   theta_1s  - Longitudinal cyclic (rad)
%   delta_E   - Elevator deflection (rad)
%
% Outputs:
%   u_lon     - [theta_0, theta_1s, delta_E]

u_lon = [theta_0, theta_1s, delta_E];

end

== matlab function Trajectory_PID/Trajectory Controller/Lateral Controller/ Course Angle ==
  data: chi output; x_E input; y_E input; x_E_ref input; y_E_ref input
function chi = Course_Angle(x_E, y_E, x_E_ref, y_E_ref)
% Author:
%   Hanchen Li (hl3422@ic.ac.uk)
%
% Inputs:
%   vx
%   vy
%
% Outputs:
%   chi_ref

chi = atan2(y_E_ref - y_E, x_E_ref - x_E);

end

== matlab function Trajectory_PID/Trajectory Controller/Lateral Controller/Transfer to Array1 ==
  data: delta_R input; u_lat output; theta_diff input; theta_1c input
function u_lat = u_lat_form(delta_R, theta_diff, theta_1c)
% Author:
%   Hanchen Li (hl3422@ic.ac.uk)
%
% Inputs:
%   theta_diff - Rotor collective difference (rad)
%   theta_1c   - Lateral cyclic (rad)
%   delta_R    - Rudder deflection (rad)
%
% Outputs:
%   u_lat      - [theta_diff, theta_1c, delta_R]

u_lat = [theta_diff, theta_1c, delta_R];

end
